simulink model "KaskadeControlled_2D"  (R2013a)
settings: Solver=ode1  StartTime=0.0  StopTime=Tend  FixedStep=t_sample  RelTol=1e-3
PreLoadFcn:
  | Control_parameter;
  | KaskadeModellInit;
PostLoadFcn:
  | , if any(exist('dsrtsu_mdlpostloadfcn', 'file') == [2, 3, 6]), try dsrtsu_mdlpostloadfcn('Execute', bdroot); catch fprintf('Error in PostLoadFcn (dsrtsu_mdlpostloadfcn) for model "%s":\n %s\n', bdroot, lasterr); end, end,
values from neighbouring files (symbols this model uses):
  alpha_0 = 0    [Control_parameter.m]
  beta_0 = 0    [Control_parameter.m]
  d_x_0 = 0    [Control_parameter.m]
  d_y_0 = 0    [Control_parameter.m]
  g = 9.81    [Control_parameter.m]    (also in KaskadeModellInit.m)
  t_sample = 0.01    [Control_parameter.m]
  x_0 = 0    [Control_parameter.m]
  y_0 = 0    [Control_parameter.m]
settings Model: DSRTSU_INTERNAL_RTI_VER=420  DSRTSU_INTERNAL_RTI_TYPE=rti1401  DSRTSU_INTERNAL_RTIFPGA=10  BufferReuse=off  Creator=Henning  LastModifiedBy=Henning
settings OptimizationCC: BlockReduction=off  OptimizeBlockIOStorage=off  BufferReuse=off  ExpressionFolding=off  LocalBlockOutputs=off
settings HardwareCC: ProdIntDivRoundTo=Zero  ProdEndianess=BigEndian  ProdHWDeviceType=Generic->Custom  TargetIntDivRoundTo=Zero  TargetEndianess=BigEndian  TargetHWDeviceType=Generic->Custom
settings RTWCC: SystemTargetFile=rti1401.tlc  MakeCommand=make_rti  TemplateMakefile=rti1401.tmf  Description=dSPACE DS1401 Hardware Platform  ProcessScript=rti1401_make_rtw_hook
settings STFCustomTargetCC: ParMdlRefBuildCompliant=on  GeneratePreprocessorConditionals=Disable all  MatFileLogging=on  GRTInterface=on  SystemTargetFile=rti1401.tlc
settings GRTTargetCC: CompOptLevelCompliant=off  ConcurrentExecutionCompliant=off  CombineOutputUpdateFcns=off  GRTInterface=on  ExtModeMexFile=noextcomm

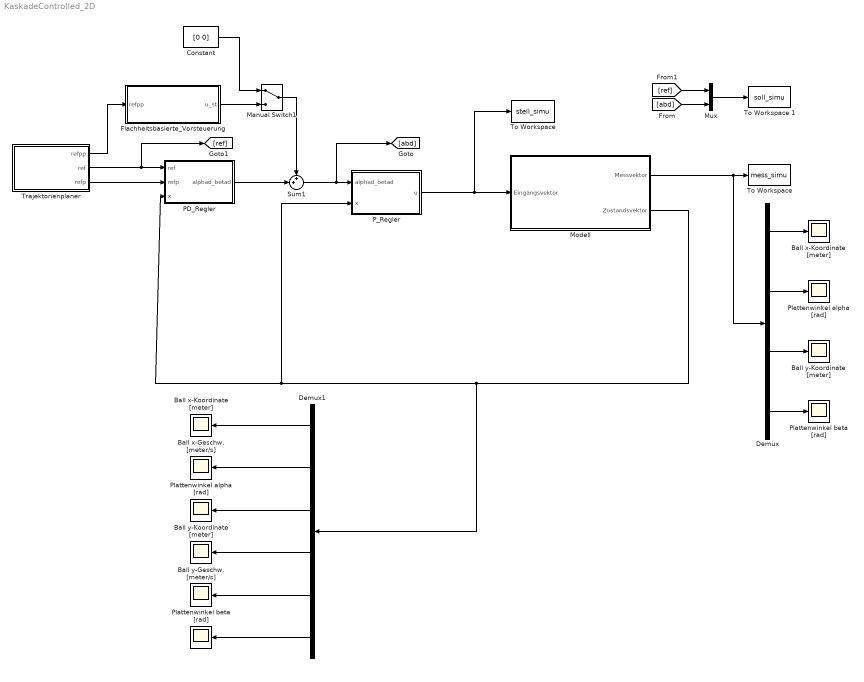
== system KaskadeControlled_2D ==
  "Ball x-Geschw. [meter/s] " : Scope
      settings: TimeRange=60  YMin=-0.4  YMax=0.3  SaveName=ScopeData2
  Ball x-Koordinate [meter] : Scope
      settings: YMin=-0.0266  YMax=-0.0251
  "Ball x-Koordinate [meter] " : Scope
      settings: YMin=0.05962  YMax=0.05983  SaveName=ScopeData5
  "Ball y-Geschw. [meter/s] " : Scope
      settings: YMin=-0.0013  YMax=0.0005  SaveName=ScopeData9
  Ball y-Koordinate [meter] : Scope
      settings: YMin=-0.175  YMax=0.2  SaveName=ScopeData3
  "Ball y-Koordinate [meter] " : Scope
      settings: YMin=-0.12425  YMax=-0.12075  SaveName=ScopeData6
  Constant : Constant  Value=[0 0]  OutDataTypeStr=boolean  SampleTime=t_sample
  Demux : Demux
  Demux1 : Demux  Outputs=6
  Flachheitsbasierte_Vorsteuerung : Subsystem
  Manual Switch1 : ManualSwitch
  Modell : Subsystem
  Mux : Mux  Inputs=2
  PD_Regler : Subsystem
  P_Regler : Subsystem
  Plattenwinkel alpha [rad] : Scope
      settings: YMin=-0.0189086  YMax=-0.0171078
  "Plattenwinkel alpha [rad] " : Scope
      settings: YMin=-1  YMax=1  SaveName=ScopeData7
  Plattenwinkel beta [rad] : Scope
      settings: YMin=-0.000258552  YMax=-0.000258552  SaveName=ScopeData4
  "Plattenwinkel beta [rad] " : Scope
      settings: SaveName=ScopeData8
  Sum1 : Sum  Inputs=++|
  To Workspace : ToWorkspace  VariableName=stell_simu  SampleTime=t_sample  SaveFormat=Structure With Time
  "To Workspace " : ToWorkspace  VariableName=mess_simu  SampleTime=t_sample  SaveFormat=Structure With Time
  To Workspace 1 : ToWorkspace  VariableName=soll_simu  SampleTime=t_sample  SaveFormat=Structure With Time
  Trajektorienplaner : Subsystem
  wires:
  Modell/1(Messvektor) -> Demux/1, "To Workspace "/1
  Demux/1 -> Ball x-Koordinate [meter]/1
  Demux/2 -> Plattenwinkel alpha [rad]/1
  Demux/3 -> Ball y-Koordinate [meter]/1
  Demux/4 -> Plattenwinkel beta [rad]/1
  Demux1/1 -> "Ball x-Koordinate [meter] "/1
  Demux1/2 -> "Ball x-Geschw. [meter/s] "/1
  Demux1/3 -> "Plattenwinkel alpha [rad] "/1
  Demux1/4 -> "Ball y-Koordinate [meter] "/1
  Demux1/5 -> "Ball y-Geschw. [meter/s] "/1
  Demux1/6 -> "Plattenwinkel beta [rad] "/1
  Modell/2(Zustandsvektor) -> Demux1/1, P_Regler/2(x), PD_Regler/3(x)
  Trajektorienplaner/2(ref) -> [ref], PD_Regler/1(ref)
  Trajektorienplaner/3(refp) -> PD_Regler/2(refp)
  Trajektorienplaner/1(refpp) -> Flachheitsbasierte_Vorsteuerung/1(refpp)
  PD_Regler/1(alphad_betad) -> Sum1/2
  Flachheitsbasierte_Vorsteuerung/1(u_st) -> Manual Switch1/2
  Constant/1 -> Manual Switch1/1
  Manual Switch1/1 -> Sum1/1
  Sum1/1 -> [abd], P_Regler/1(alphad_betad)
  P_Regler/1(u) -> To Workspace/1, Modell/1(Eingangsvektor)
  Mux/1 -> To Workspace 1/1
  [abd] -> Mux/2
  [ref] -> Mux/1

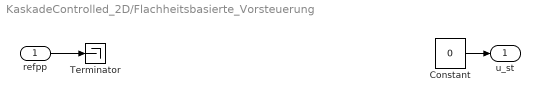
== system KaskadeControlled_2D/Flachheitsbasierte_Vorsteuerung ==
  refpp : Inport
  Constant : Constant  Value=0
  Terminator : Terminator
  u_st : Outport
  wires:
  refpp/1 -> Terminator/1
  Constant/1 -> u_st/1

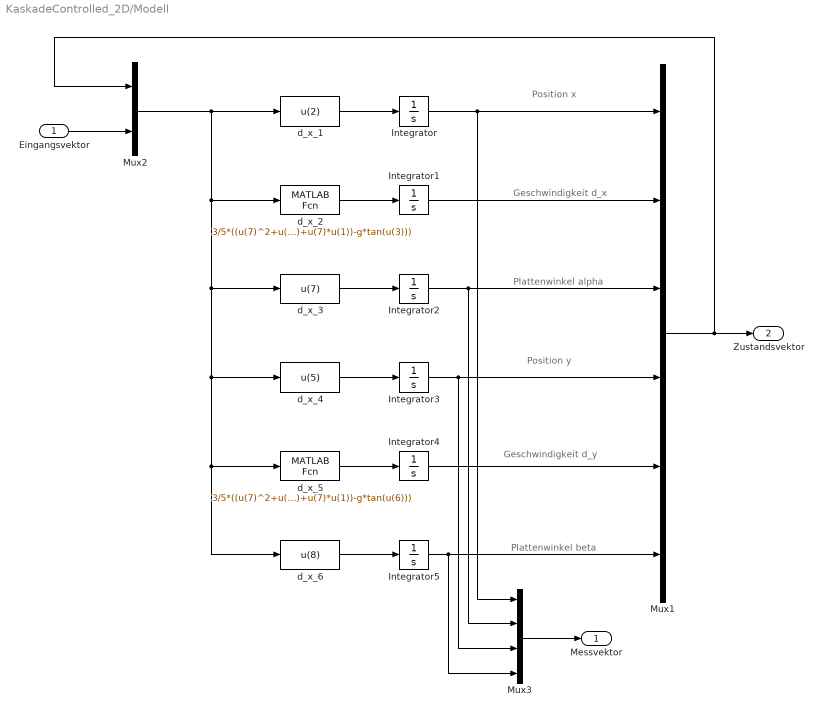
== system KaskadeControlled_2D/Modell ==
  note: Position x
  note: Geschwindigkeit d_x
  note: Plattenwinkel alpha
  note: Position y
  note: Geschwindigkeit d_y
  note: Plattenwinkel beta
  Eingangsvektor : Inport
  Integrator : Integrator  InitialCondition=x_0
  Integrator1 : Integrator  InitialCondition=d_x_0
  Integrator2 : Integrator  InitialCondition=alpha_0
  Integrator3 : Integrator  InitialCondition=y_0
  Integrator4 : Integrator  InitialCondition=d_y_0
  Integrator5 : Integrator  InitialCondition=beta_0
  Mux1 : Mux  Inputs=6
  Mux2 : Mux  Inputs=2
  Mux3 : Mux
  d_x_1 : MATLABFcn  MATLABFcn=u(2)
  d_x_2 : MATLABFcn  MATLABFcn=3/5*((u(7)^2+u(8)^2)*tan(u(3))*(u(1)*tan(u(3))+u(4)*tan(u(6)))+u(7)*(u(8)*u(4)+u(7)*u(1))-g*tan(u(3)))
  d_x_3 : MATLABFcn  MATLABFcn=u(7)
  d_x_4 : MATLABFcn  MATLABFcn=u(5)
  d_x_5 : MATLABFcn  MATLABFcn=3/5*((u(7)^2+u(8)^2)*tan(u(6))*(u(1)*tan(u(3))+u(4)*tan(u(6)))+u(8)*(u(8)*u(4)+u(7)*u(1))-g*tan(u(6)))
  d_x_6 : MATLABFcn  MATLABFcn=u(8)
  Messvektor : Outport
  Zustandsvektor : Outport  Port=2
  wires:
  Eingangsvektor/1 -> Mux2/2
  d_x_1/1 -> Integrator/1
  d_x_2/1 -> Integrator1/1
  d_x_3/1 -> Integrator2/1
  d_x_4/1 -> Integrator3/1
  d_x_5/1 -> Integrator4/1
  d_x_6/1 -> Integrator5/1
  Mux1/1 -> Zustandsvektor/1, Mux2/1
  Mux2/1 -> d_x_1/1, d_x_3/1, d_x_5/1, d_x_6/1, d_x_4/1, d_x_2/1
  Mux3/1 -> Messvektor/1
  Integrator/1 -> Mux1/1, Mux3/1
  Integrator1/1 -> Mux1/2
  Integrator2/1 -> Mux1/3, Mux3/2
  Integrator3/1 -> Mux1/4, Mux3/3
  Integrator4/1 -> Mux1/5
  Integrator5/1 -> Mux1/6, Mux3/4

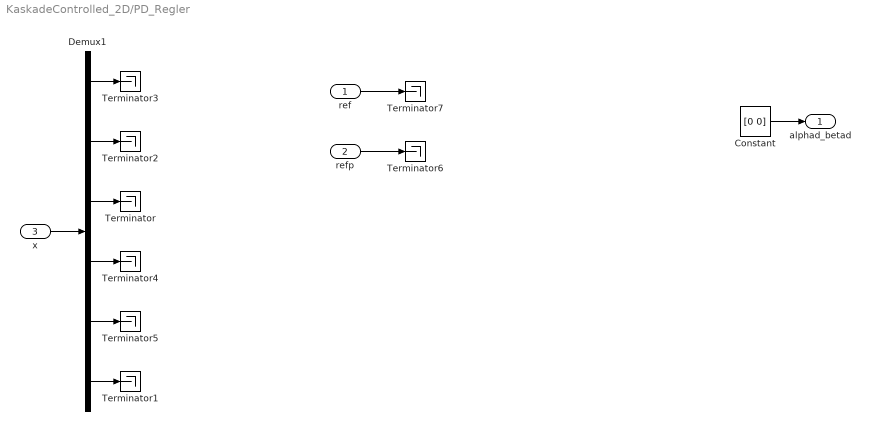
== system KaskadeControlled_2D/PD_Regler ==
  ref : Inport
  refp : Inport  Port=2
  x : Inport  Port=3
  Constant : Constant  Value=[0 0]
  Demux1 : Demux  Outputs=6
  Terminator{,1..7} (8 alike) : Terminator
  alphad_betad : Outport
  wires:
  x/1 -> Demux1/1
  Demux1/3 -> Terminator/1
  Demux1/6 -> Terminator1/1
  Demux1/1 -> Terminator3/1
  Demux1/2 -> Terminator2/1
  Demux1/5 -> Terminator5/1
  Demux1/4 -> Terminator4/1
  refp/1 -> Terminator6/1
  ref/1 -> Terminator7/1
  Constant/1 -> alphad_betad/1

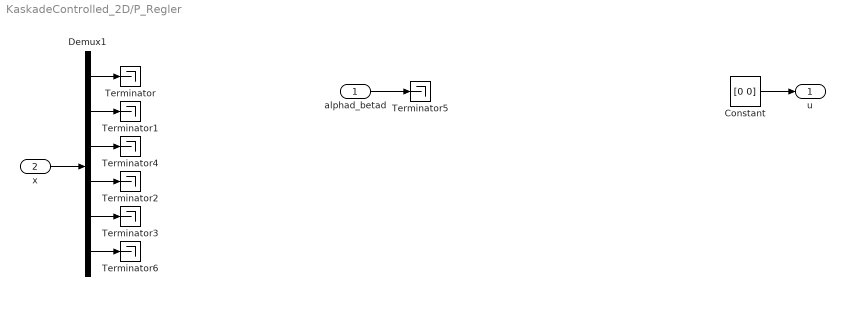
== system KaskadeControlled_2D/P_Regler ==
  alphad_betad : Inport
  x : Inport  Port=2
  Constant : Constant  Value=[0 0]
  Demux1 : Demux  Outputs=6
  Terminator{,1..6} (7 alike) : Terminator
  u : Outport
  wires:
  x/1 -> Demux1/1
  Demux1/2 -> Terminator1/1
  Demux1/1 -> Terminator/1
  Demux1/4 -> Terminator2/1
  Demux1/5 -> Terminator3/1
  alphad_betad/1 -> Terminator5/1
  Demux1/6 -> Terminator6/1
  Demux1/3 -> Terminator4/1
  Constant/1 -> u/1

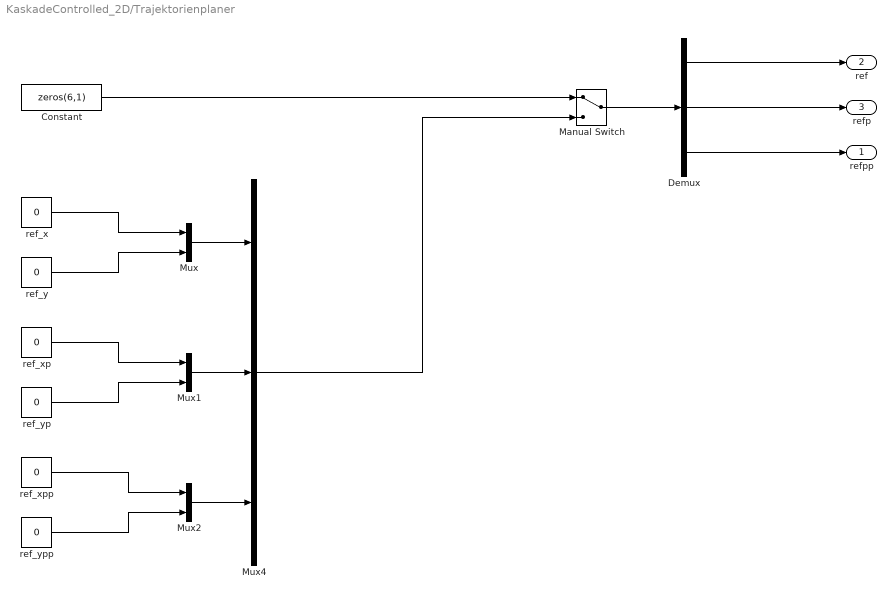
== system KaskadeControlled_2D/Trajektorienplaner ==
  Constant : Constant  Value=zeros(6,1)  SampleTime=t_sample
  Demux : Demux  Outputs=3
  Manual Switch : ManualSwitch
  Mux : Mux  Inputs=2
  Mux1 : Mux  Inputs=2
  Mux2 : Mux  Inputs=2
  Mux4 : Mux  Inputs=3
  ref_x : Constant  Value=0
  ref_xp : Constant  Value=0
  ref_xpp : Constant  Value=0
  ref_y : Constant  Value=0
  ref_yp : Constant  Value=0
  ref_ypp : Constant  Value=0
  refpp : Outport
  ref : Outport  Port=2
  refp : Outport  Port=3
  wires:
  ref_y/1 -> Mux/2
  ref_x/1 -> Mux/1
  ref_yp/1 -> Mux1/2
  ref_xp/1 -> Mux1/1
  Constant/1 -> Manual Switch/1
  Mux/1 -> Mux4/1
  Mux1/1 -> Mux4/2
  Mux2/1 -> Mux4/3
  Manual Switch/1 -> Demux/1
  Mux4/1 -> Manual Switch/2
  Demux/1 -> ref/1
  Demux/2 -> refp/1
  Demux/3 -> refpp/1
  ref_xpp/1 -> Mux2/1
  ref_ypp/1 -> Mux2/2
